simulink model "P_model"  (R2020b)
settings: Solver=VariableStepAuto  StartTime=0.0  StopTime=50  MaxStep=0.0001  RelTol=1e-3
settings Model: Creator=valerio  LastModifiedBy=simon

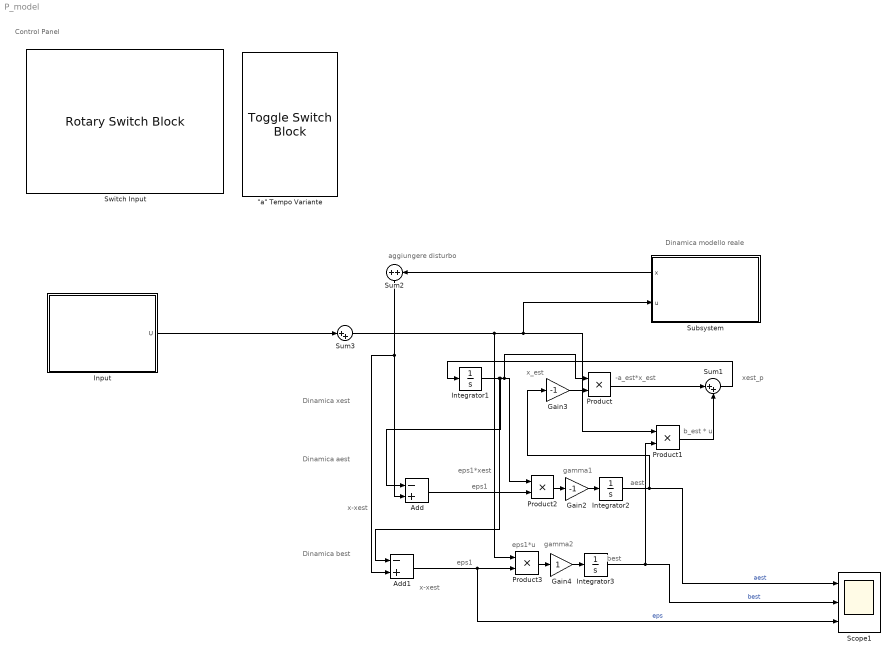
== system P_model ==
  note: Control Panel
  note: eps1*xest
  note: eps1*u
  note: gamma2
  note: gamma1
  note: x-xest
  note: aggiungere disturbo
  note: eps1
  note: eps1
  note: best
  note: Dinamica best
  note: aest
  note: Dinamica aest
  note: Dinamica modello reale
  note: Dinamica xest
  note: x_est
  note: -a_est*x_est
  note: b_est * u
  note: xest_p
  note: x-xest
  " \"a\" Tempo Variante" : ToggleSwitchBlock  LabelPosition=Hide
      settings: Values={{'Off', 'On'}, [1 2]}
  Add : Sum  Inputs=-+
  Add1 : Sum  Inputs=-+
  Gain2 : Gain  Gain=-1
  Gain3 : Gain  Gain=-1
  Gain4 : Gain
  Input : Subsystem
  Integrator1 : Integrator
  Integrator2 : Integrator
  Integrator3 : Integrator
  Product{,1..3} (4 alike) : Product
  Scope1 : Scope  NumInputPorts=3
  Subsystem : Subsystem
      settings: PortSchema="{\"entries\":[{\"content\":{\"sides\":[{\"content\":{\"connectorIds\":[\"Out1\",\"In1\"]},\"type\":\"ConnectorPlacement.EquallySpacedRectSide\",\"uuid\":\"29482476-401b-41e7-9ad6-c6af3f7ca46f\"},{\"content\":{\"connectorIds\":[],\"side\":\"RIGHT\"},\"type\":\"ConnectorPlacement.EquallySpacedRectSide\",\"uuid\":\"f6eae66b-0fdb-4798-98ce-b6245a6528d3\"},{\"content\":{\"connectorIds\":[],\"side\":\"TOP\"},\"type\":\"ConnectorPlacement.EquallySpacedRectSide\",\"uuid\":\"bf44f428-fe33-46a7-93c0-690038f41b99\"}]},\"type\":\"ConnectorPlacement.EquallySpacedConnector\",\"uuid\":\"07e71849-cf32-484a-a28b-980fa66d4ee9\"}],\"packageUris\":[\"http://schema.mathworks.com/mf0/Connector/R2020b\"],\"version\":\"1.0\"}"
  Sum1 : Sum  Inputs=|++
  Sum2 : Sum  Inputs=+|+
  Sum3 : Sum  Inputs=|++
  Switch Input : RotarySwitchBlock  LabelPosition=Hide
      settings: Values={{'sin', 'step', 'cost'}, [1 2 3]}
  wires:
  Integrator1/1 -> Product2/1, Product/1, Add/1, Add1/1
  Product/1 -> Sum1/1
  Sum1/1 -> Integrator1/1
  Product1/1 -> Sum1/2
  Product2/1 -> Gain2/1
  Gain2/1 -> Integrator2/1
  Add/1 -> Product2/2
  Add1/1 -> Scope1/3, Product3/2  "eps"
  Product3/1 -> Gain4/1
  Integrator3/1 -> Scope1/2, Product1/2  "best"
  Integrator2/1 -> Scope1/1, Gain3/1  "aest"
  Gain3/1 -> Product/2
  Sum2/1 -> Add1/2, Add/2
  Gain4/1 -> Integrator3/1
  Sum3/1 -> Product1/1, Subsystem/1(u), Product3/1
  Subsystem/1(x) -> Sum2/2
  Input/1(U) -> Sum3/1

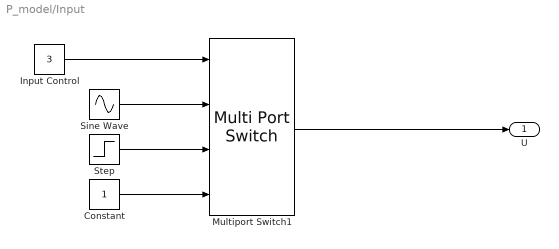
== system P_model/Input ==
  Constant : Constant
  Input Control : Constant  Value=3
  Multiport Switch1 : MultiPortSwitch
  Sine Wave : Sin  SampleTime=0
  Step : Step  SampleTime=0
  U : Outport
  wires:
  Input Control/1 -> Multiport Switch1/1
  Step/1 -> Multiport Switch1/3
  Constant/1 -> Multiport Switch1/4
  Sine Wave/1 -> Multiport Switch1/2
  Multiport Switch1/1 -> U/1

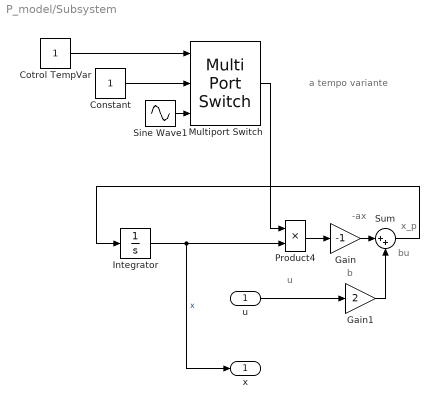
== system P_model/Subsystem ==
  note: a tempo variante
  note: b
  note: bu
  note: -ax
  note: x_p
  note: u
  u : Inport
  Constant : Constant
  Cotrol TempVar : Constant
  Gain : Gain  Gain=-1
  Gain1 : Gain  Gain=2
  Integrator : Integrator
  Multiport Switch : MultiPortSwitch  Inputs=2
  Product4 : Product
  Sine Wave1 : Sin  Bias=1  Frequency=2*pi/(24*3600)  SampleTime=0
  Sum : Sum  Inputs=|++
  x : Outport
  wires:
  Gain/1 -> Sum/1
  Sum/1 -> Integrator/1
  Gain1/1 -> Sum/2
  Integrator/1 -> Product4/2, x/1  "x"
  u/1 -> Gain1/1
  Product4/1 -> Gain/1
  Multiport Switch/1 -> Product4/1
  Cotrol TempVar/1 -> Multiport Switch/1
  Constant/1 -> Multiport Switch/2
  Sine Wave1/1 -> Multiport Switch/3
